simulink model "PID_model_reference"  (R2020b)
settings: Solver=VariableStepAuto  StartTime=0.0  StopTime=10.0  RelTol=1e-3
undefined symbols (not defined in the file or in its folder): Kd, Ki, Kp
settings Model: DataDictionary=dict.sldd  Creator=Sudhanshu  LastModifiedBy=Sudhanshu
settings DataIOCC: SaveOutput=off  SaveTime=off

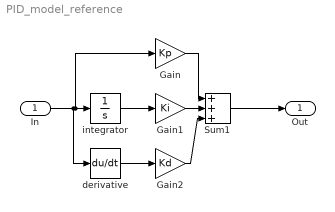
== system PID_model_reference ==
  In : Inport  OutDataTypeStr=double  PortDimensions=1  SampleTime=0
  Gain : Gain  Gain=Kp
  Gain1 : Gain  Gain=Ki
  Gain2 : Gain  Gain=Kd
  Sum1 : Sum  Inputs=+++
  derivative : Derivative
  integrator : Integrator
  Out : Outport  OutDataTypeStr=double  PortDimensions=1  SampleTime=0
  wires:
  Gain1/1 -> Sum1/2
  Gain2/1 -> Sum1/3
  Gain/1 -> Sum1/1
  In/1 -> integrator/1, Gain/1, derivative/1
  derivative/1 -> Gain2/1
  integrator/1 -> Gain1/1
  Sum1/1 -> Out/1
